simulink model "minor"  (R2023b)
settings: Solver=VariableStepAuto  StartTime=0.0  StopTime=10.0  RelTol=1e-3
settings Model: Creator=Spedrik Webster  LastModifiedBy=Avijeet Jain

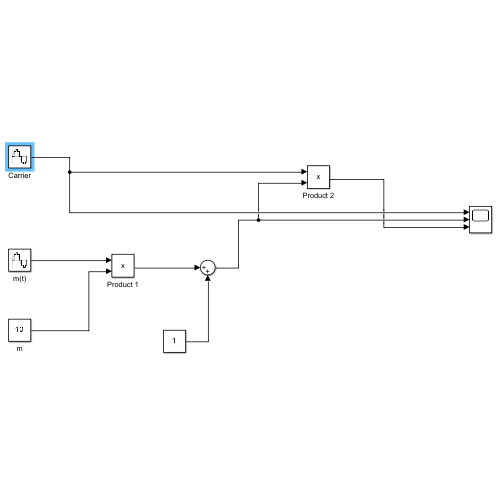
[thumbnail: Simulink's stored preview of the top-level diagram]
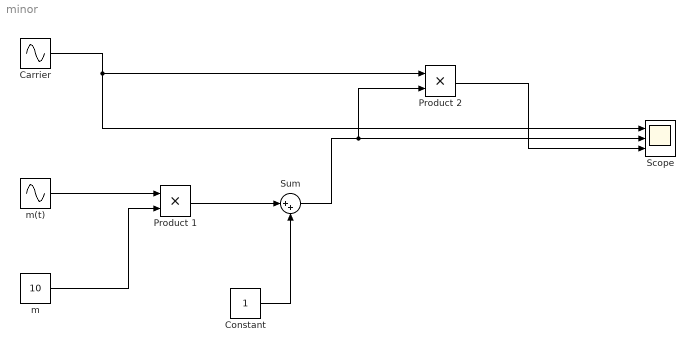
== system minor ==
  Carrier : Sin  Amplitude=3  Frequency=500  SampleTime=1/5000
  Constant : Constant
  Product 1 : Product
  Product 2 : Product
  Scope : Scope  NumInputPorts=3
  Sum : Sum  Inputs=|++
  m : Constant  Value=10
  m(t) : Sin  Amplitude=3  Frequency=50  SampleTime=1/5000
  wires:
  Carrier/1 -> Product 2/1, Scope/1
  m(t)/1 -> Product 1/1
  Product 1/1 -> Sum/1
  m/1 -> Product 1/2
  Sum/1 -> Scope/2, Product 2/2
  Product 2/1 -> Scope/3
  Constant/1 -> Sum/2
